simulink model "DC_motor"  (R2013b)
settings: Solver=ode45  StartTime=0.0  StopTime=90  MaxStep=0.1  RelTol=1e-3
values from neighbouring files (symbols this model uses):
  J = 1.66e-5    (= 1.66e-05)    [RunMotorSim.m]    (also in RunMotorSim_OpenLoop.m)
  KD = 1.33e-8    (= 1.33e-08)    [RunMotorSim.m]    (also in RunMotorSim_OpenLoop.m)
  KT = 7.5e-3    (= 0.0075)    [RunMotorSim.m]    (also in RunMotorSim_OpenLoop.m)
  pow = 1.88    [RunMotorSim.m]    (also in RunMotorSim_OpenLoop.m = 2)
settings Model: Creator=aberger  LastModifiedBy=aberger

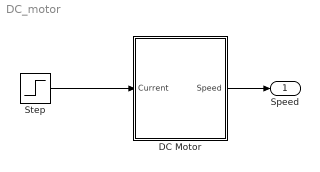
== system DC_motor ==
  DC Motor : Subsystem
  Step : Step  Time=0  After=0.27  SampleTime=0
  Speed : Outport
  wires:
  Step/1 -> DC Motor/1(Current)
  DC Motor/1(Speed) -> Speed/1

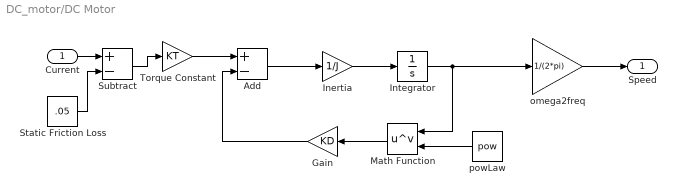
== system DC_motor/DC Motor ==
  Current : Inport
  Add : Sum  Inputs=+-
  Gain : Gain  Gain=KD
  Inertia : Gain  Gain=1/J
  Integrator : Integrator
  Math Function : Math  Operator=pow  SaturateOnIntegerOverflow=on
  Static Friction Loss : Constant  Value=.05
  Subtract : Sum  Inputs=+-
  Torque Constant : Gain  Gain=KT
  omega2freq : Gain  Gain=1/(2*pi)
  powLaw : Constant  Value=pow
  Speed : Outport
  wires:
  Add/1 -> Inertia/1
  Integrator/1 -> Math Function/1, omega2freq/1
  Torque Constant/1 -> Add/1
  Gain/1 -> Add/2
  Inertia/1 -> Integrator/1
  Current/1 -> Subtract/1
  Math Function/1 -> Gain/1
  omega2freq/1 -> Speed/1
  Subtract/1 -> Torque Constant/1
  Static Friction Loss/1 -> Subtract/2
  powLaw/1 -> Math Function/2
